simulink model "PD_control"  (R2023b)
settings: Solver=VariableStepAuto  StartTime=0.0  StopTime=20  RelTol=1e-3
values from neighbouring files (symbols this model uses):
  ctrl_gains = [1.75;1.75;1.75;6;6;6]    [quadcopterMain.m]
  param = [Ixx;Iyy;Izz;l;k;b;m]    [main_matteo.m]    (also in quadcopterMain.m)
  Ts_slk = 0.01    [main_matteo.m]    (also in quadcopterMain.m)
  x_des = [10;12;10;15;20;25]    [quadcopterMain.m]
  x_eq = [0;0;0;0;0;0]    [main_matteo.m]    (also in quadcopterMain.m)
settings Model: Creator=asus  LastModifiedBy=asus
settings OptimizationCC: ReuseModelBlockBuffer=off

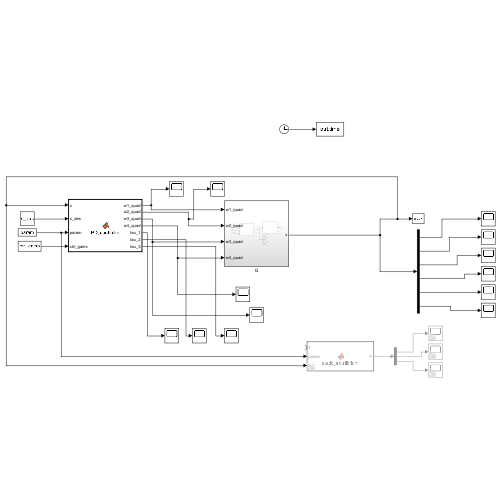
[thumbnail: Simulink's stored preview of the top-level diagram]
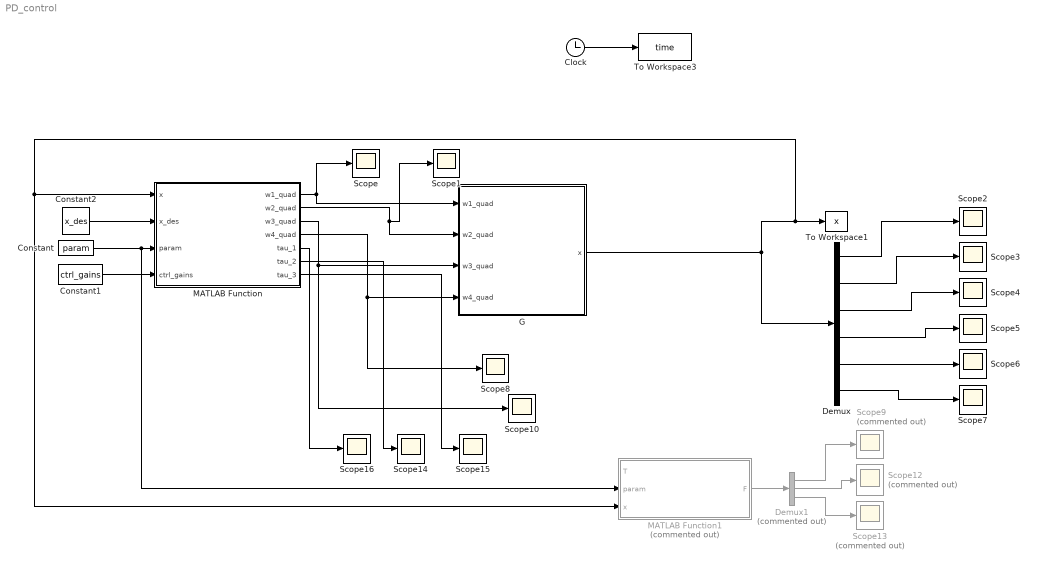
== system PD_control ==
  Clock : Clock
  Constant : Constant  Value=param
  Constant1 : Constant  Value=ctrl_gains
  Constant2 : Constant  Value=x_des
  Demux : Demux  Outputs=6
  Demux1 : Demux  Commented=on  Outputs=3
  G : Subsystem
  MATLAB Function : MATLAB Function  TreatAsAtomicUnit=on
  MATLAB Function1 : MATLAB Function  Commented=on  TreatAsAtomicUnit=on
  Scope{,1..8,10,14..16} (13 alike) : Scope
  Scope12 : Scope  Commented=on
  Scope13 : Scope  Commented=on
  Scope9 : Scope  Commented=on
  To Workspace1 : ToWorkspace  VariableName=x  SampleTime=-1
      settings: Save2DSignal=2-D array (concatenate along first dimension)
  To Workspace3 : ToWorkspace  VariableName=time  SampleTime=Ts_slk
      settings: Save2DSignal=2-D array (concatenate along first dimension)
  wires:
  Clock/1 -> To Workspace3/1
  Constant1/1 -> MATLAB Function/4(ctrl_gains)
  Constant/1 -> MATLAB Function1/2(param), MATLAB Function/3(param)
  Demux/3 -> Scope4/1
  Demux/1 -> Scope2/1
  Demux/4 -> Scope5/1
  Demux/6 -> Scope7/1
  Demux/2 -> Scope3/1
  Demux/5 -> Scope6/1
  Constant2/1 -> MATLAB Function/2(x_des)
  MATLAB Function1/1(F) -> Demux1/1
  Demux1/1 -> Scope9/1
  Demux1/2 -> Scope12/1
  Demux1/3 -> Scope13/1
  G/1(x) -> MATLAB Function1/3(x), MATLAB Function/1(x), To Workspace1/1, Demux/1
  MATLAB Function/1(w1_quad) -> G/1(w1_quad), Scope/1
  MATLAB Function/2(w2_quad) -> Scope1/1, G/2(w2_quad)
  MATLAB Function/3(w3_quad) -> Scope10/1, G/3(w3_quad)
  MATLAB Function/4(w4_quad) -> Scope8/1, G/4(w4_quad)
  MATLAB Function/5(tau_1) -> Scope16/1
  MATLAB Function/6(tau_2) -> Scope14/1
  MATLAB Function/7(tau_3) -> Scope15/1

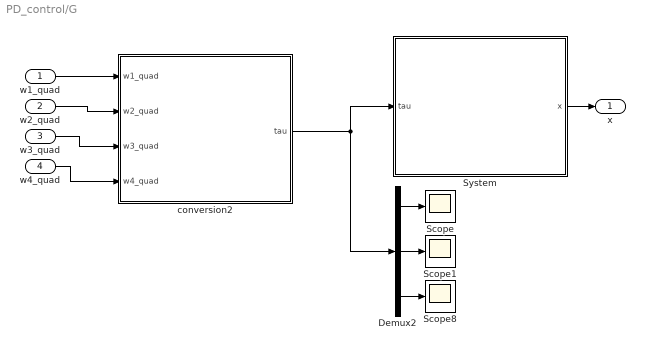
== system PD_control/G ==
  w1_quad : Inport
  w2_quad : Inport  Port=2
  w3_quad : Inport  Port=3
  w4_quad : Inport  Port=4
  Demux2 : Demux  Outputs=3
  Scope : Scope
  Scope1 : Scope
  Scope8 : Scope
  System : Subsystem
  conversion2 : Subsystem
  x : Outport
  wires:
  w4_quad/1 -> conversion2/4(w4_quad)
  Demux2/2 -> Scope1/1
  Demux2/3 -> Scope8/1
  Demux2/1 -> Scope/1
  System/1(x) -> x/1
  conversion2/1(tau) -> System/1("tau "), Demux2/1
  w1_quad/1 -> conversion2/1(w1_quad)
  w2_quad/1 -> conversion2/2(w2_quad)
  w3_quad/1 -> conversion2/3(w3_quad)

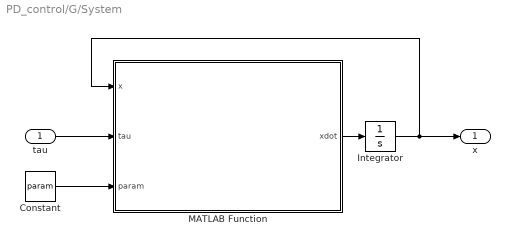
== system PD_control/G/System ==
  "tau " : Inport
  Constant : Constant  Value=param
  Integrator : Integrator  InitialCondition=x_eq
  MATLAB Function : MATLAB Function  TreatAsAtomicUnit=on
  x : Outport
  wires:
  Integrator/1 -> MATLAB Function/1(x), x/1
  MATLAB Function/1(xdot) -> Integrator/1
  "tau "/1 -> MATLAB Function/2(tau)
  Constant/1 -> MATLAB Function/3(param)

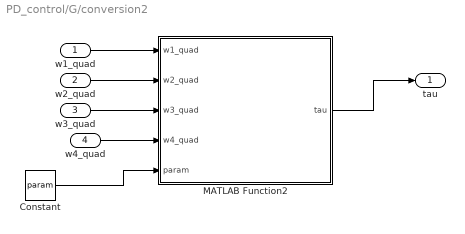
== system PD_control/G/conversion2 ==
  w1_quad : Inport
  w2_quad : Inport  Port=2
  w3_quad : Inport  Port=3
  w4_quad : Inport  Port=4
  Constant : Constant  Value=param
  MATLAB Function2 : MATLAB Function  TreatAsAtomicUnit=on
  tau : Outport
  wires:
  MATLAB Function2/1(tau) -> tau/1
  w4_quad/1 -> MATLAB Function2/4(w4_quad)
  w3_quad/1 -> MATLAB Function2/3(w3_quad)
  Constant/1 -> MATLAB Function2/5(param)
  w1_quad/1 -> MATLAB Function2/1(w1_quad)
  w2_quad/1 -> MATLAB Function2/2(w2_quad)

== matlab function PD_control/G/System/MATLAB Function ==
  data: x input; tau input; xdot output; param input
function xdot=quadcopter(x,tau,param)
% Inputs:
%           x       (model state)
%           tau     (torque)           
%           param   (model parameters)
%
% Outputs:  x_dot  (derivative of the state with respect to time)

% Import roll, pitch, yaw accelerations
% Parameters
g        =       9.81;           %  gravity acceleration (m/s^2)
Ixx      =       param(1,1);     %  moment of inertia 
Iyy      =       param(2,1);     %  moment of inertia
Izz      =       param(3,1);     %  moment of inertia 

% States
phi      =       x(1,1);     %  roll angle (rad)
theta    =       x(2,1);     %  pitch angle (rad)
psi      =       x(3,1);     %  yaw angle (rad)  
phi_dot  =       x(4,1);     %  roll rate (rad/s)
theta_dot=       x(5,1);     %  pitch rate (rad/s)
psi_dot  =       x(6,1);     %  yaw rate (rad/s)  

cph         =       cos(phi);
cth         =       cos(theta);
cps         =       cos(psi);
sph         =       sin(phi);
sth         =       sin(theta);
sps         =       sin(psi);

% torques
tau_1    =       tau(1,1);   %  roll torque 
tau_2    =       tau(2,1);   %  pitch torque 
tau_3    =       tau(3,1);   %  yaw torque   

% Coriolis matrix
C11=  0;
C12= (Iyy-Izz)*(theta_dot*cph*sph+psi_dot*sph^2*cth)+(Izz-Iyy)*psi_dot*cph^2*cth-Ixx*psi_dot*cth;
C13= (Izz-Iyy)*psi_dot*cph*sph*cth^2;
C21= (Izz-Iyy)*(theta_dot*cph*sph+psi_dot*sph*cth)+(Iyy-Izz)*psi_dot*cph^2*cth+Ixx*psi_dot*cth;
C22= (Izz-Iyy)*psi_dot*cph*sph;
C23= -Ixx*psi_dot*sth*cth+Iyy*psi_dot*sph^2*sth*cth+Izz*psi_dot*cph^2*sth*cth;
C31= (Iyy-Izz)*psi_dot*cth^2*sph*cph-Ixx*theta_dot*cth;
C32= (Izz-Iyy)*(theta_dot*cph*sph*sth+phi_dot*sph^2*cth)+(Iyy-Izz)*phi_dot*cph^2*cth+Ixx*psi_dot*sth*cth-Iyy*psi_dot*sph^2*sth*cth-Izz*psi_dot*cph^2*sth*cth;
C33= (Iyy-Izz)*phi_dot*cph*sph*cth^2-Iyy*theta_dot*sph^2*cth*sth-Izz*theta_dot*cph^2*cth*sth+Ixx*theta_dot*cth*sth;

C  = [C11 C12 C13;
    C21 C22 C23;
    C31 C32 C33];

% Inertia matrix
J11= Ixx;
J12= 0;
J13= -Ixx*sth;
J21= 0;
J22= Iyy*cph^2+Izz*sph^2;
J23= (Iyy-Izz)*cph*sph*cth;
J31= -Ixx*sth;
J32= (Iyy-Izz)*cph*sph*cth;
J33= Ixx*sth^2+Iyy*sph^2*cth^2+Izz*cph^2*cth^2;

J  = [J11 J12 J13;
    J21 J22 J23;
    J31 J32 J33];
%% Model equations
A          = C11*phi_dot+C12*theta_dot+C13*psi_dot;
B          = C21*phi_dot+C22*theta_dot+C23*psi_dot;
M          = C31*phi_dot+C32*theta_dot+C33*psi_dot;
H          = J11*(tau(3,1)-M)-J31*(tau(1,1)-A);
E          = (J32*J11-J31*J12)/(J11*J22-J21*J12);
D          = (tau(2,1)-B)*J11-(tau(1,1)-A)*J21;
F          = J11*J23-J21*J13;
L          = J33*J11-J31*J13;

xdot       = zeros(6,1);
xdot(1,1)  = phi_dot;
xdot(2,1)  = theta_dot;  
xdot(3,1)  = psi_dot;
xdot(4,1)  = ((tau(1,1)-A)-J12*(D-F*((H-E*D)/(L-E*F)))-J13*((H-E*D)/(L-E*F)))/J11;
xdot(5,1)  = D-F*((H-E*D)/(L-E*F));
xdot(6,1)  = (H-E*D)/(L-E*F);

== matlab function PD_control/MATLAB Function ==
  data: x input; w1_quad output; x_des input; param input; w2_quad output; ctrl_gains input; w3_quad output; w4_quad output; tau_1 output; tau_2 output; tau_3 output
function [w1_quad,w2_quad,w3_quad,w4_quad, tau_1, tau_2,tau_3] = PD_controller(x,x_des,param,ctrl_gains)
% Inputs:
%           x       (model state)
%           x_des   (desired state)           
%           param   (model parameters)
%           ctrl_gains (control gains)
%
% Outputs:  
%           wi_quad     (square of i-th propeller angular velocity)


% Parameters
g        =       9.81;           %  gravity acceleration (m/s^2)
Ixx      =       param(1,1);     %  moment of inertia 
Iyy      =       param(2,1);     %  moment of inertia
Izz      =       param(3,1);     %  moment of inertia
l        =       param(4,1);     %  //TODO da stimare   
k        =       param(5,1);     %  //TODO da stimare
b        =       param(6,1);     %  //TODO da stimare
m        =       param(7,1);     %  mass (kg)

% States
phi      =       x(1,1);     %  roll angle (rad)
theta    =       x(2,1);     %  pitch angle (rad)
psi      =       x(3,1);     %  yaw angle (rad)  
phi_dot  =       x(4,1);     %  roll rate (rad/s)
theta_dot=       x(5,1);     %  pitch rate (rad/s)
psi_dot  =       x(6,1);     %  yaw rate (rad/s)  

% Target states
phi_des      =       x_des(1,1);     %  target roll angle (rad)
theta_des    =       x_des(2,1);     %  target pitch angle (rad)
psi_des      =       x_des(3,1);     %  target yaw angle (rad)  
phi_dot_des  =       x_des(4,1);     %  target roll rate (rad/s)
theta_dot_des=       x_des(5,1);     %  target pitch rate (rad/s)
psi_dot_des  =       x_des(6,1);     %  target yaw rate (rad/s) 

% Control gains
K_ph_d      =       ctrl_gains(1,1);
K_th_d      =       ctrl_gains(2,1);
K_ps_d      =       ctrl_gains(3,1);
K_ph_p      =       ctrl_gains(4,1);
K_th_p      =       ctrl_gains(5,1);
K_ps_p      =       ctrl_gains(6,1);

% Control
tau_1       =       Ixx*(K_ph_d*(phi_dot_des-phi_dot)+K_ph_p*(phi_des-phi));
tau_2       =       Iyy*(K_th_d*(theta_dot_des-theta_dot)+K_th_p*(theta_des-theta));
tau_3       =       Izz*(K_ps_d*(psi_dot_des-psi_dot)+K_ps_p*(psi_des-psi));

cph         =       cos(phi);
cth         =       cos(theta);
T           =       m*g/cth/cph;

w1_quad     =       T/(4*k)-tau_2/(2*k*l)-tau_3/(4*b);        % w1^2
w2_quad     =       T/(4*k)-tau_1/(2*k*l)+tau_3/(4*b);
w3_quad     =       T/(4*k)+tau_2/(2*k*l)-tau_3/(4*b);
w4_quad     =       T/(4*k)+tau_1/(2*k*l)+tau_3/(4*b);

== matlab function PD_control/MATLAB Function1 ==
  data: T input; F output; param input; x input
function F = static_equilibrium(T,param,x)
% Inputs:   
%           x       (model state)
%           param   (model parameters) 
%           T       (thrust)
%
% Outputs:  F       (force constraint)


% scrivere dinamica lineare
g        =       9.81;           %  gravity acceleration (m/s^2)
m        =       param(7,1);     %  mass (kg)

phi      =       x(1,1);     %  roll angle (rad)
theta    =       x(2,1);     %  pitch angle (rad)
psi      =       x(3,1);     %  yaw angle (rad)  

cph         =       cos(phi);
cth         =       cos(theta);
cps         =       cos(psi);
sph         =       sin(phi);
sth         =       sin(theta);
sps         =       sin(psi);

R       =       [cps*sth*cph+sps*sph;
                  sps*sth*cph-cps*sph;
                  cth*cph];
G       =       g*[0;0;1];
F       =       R*T-m*G;

== matlab function PD_control/G/conversion2/MATLAB Function2 ==
  data: w1_quad input; tau output; w2_quad input; w3_quad input; w4_quad input; param input
function tau   =conversion_2(w1_quad,w2_quad,w3_quad,w4_quad,param)
% Inputs:   
%           wi_quad  (angular velocity of propeller i square)
%           param   (model parameters)   
%
% Outputs:  
%           tau     (torque)
%           T       (thrust)


% Parameters
g         =       9.81;         %  gravity acceleration (m/s^2)
l         =       param(4,1);   %  //TODO da stimare   
k         =       param(5,1);   %  //TODO da stimare
b         =       param(6,1);   %  //TODO da stimare
m         =       param(7,1);   %  mass (kg)

% motor torques
% tau_m     =       zeros(4,1);
tau_m1    =       b*w1_quad;   %  torque motor 1
tau_m2    =       b*w2_quad;   %  torque motor 2
tau_m3    =       b*w3_quad;   %  torque motor 3  
tau_m4    =       b*w4_quad;   %  torque motor 4
% 
% T         =       k*(w1_quad+w2_quad+w3_quad+w4_quad);

% torques
tau       =       zeros(3,1);
tau(1,1)  =       l*k*(-w2_quad+w4_quad); % TODO //da sistemare in base ai numeri dei motori reali
tau(2,1)  =       l*k*(-w1_quad+w3_quad);
tau(3,1)  =       -tau_m1+tau_m2-tau_m3+tau_m4;
